simulink model "WindTurbineModel_V2"  (R2025b)
settings: Solver=FixedStepDiscrete  StartTime=0.0  StopTime=inf  FixedStep=.00011  RelTol=1e-3  EnableMultiTasking=on
model workspace (MAT data in the model file):
  lambda = 10
  rho = 1.125
libraries: simulink x4, arduinolib x2, arduinosensorlib x1, slpidlib x1
settings Model: SimulationMode=external  ExtModeTrigDuration=2  Creator=Patron  LastModifiedBy=WEI
settings SolverCC: AllowMultiTaskInputOutput=on  ConcurrentTasks=on  AlgebraicLoopSolver=TrustRegion  AutoInsertRateTranBlk=on  DecoupledContinuousIntegration=on  MinimalZcImpactIntegration=on
settings DataIOCC: ReturnWorkspaceOutputs=off
settings OptimizationCC: EnhancedBackFolding=on  BooleansAsBitfields=on  PassReuseOutputArgsAs=Individual arguments  StateBitsets=on  DataBitsets=on  ZeroExternalMemoryAtStartup=off  ZeroInternalMemoryAtStartup=off  MaxStackSize=64  DifferentSizesBufferReuse=on  OptimizationPriority=RAM  OptimizationCustomize=off  EfficientTunableParamExpr=on
settings DebuggingCC: ParameterTunabilityLossMsg=error  UnconnectedInputMsg=warning  UnconnectedOutputMsg=warning  UnconnectedLineMsg=warning  ArithmeticOperatorsInVariantConditions=warning
settings HardwareCC: ProdBitPerInt=16.0  ProdBitPerPointer=16.0  ProdBitPerSizeT=16.0  ProdBitPerPtrDiffT=16.0  ProdLargestAtomicFloat=None  ProdWordSize=8.0  ProdHWDeviceType=Atmel->AVR
settings ModelReferenceCC: EnableRefExpFcnMdlSchedulingChecks=on
settings SFSimCC: SimUseLocalCustomCode=off  MATLABDynamicMemAlloc=off  CustomCodeUndefinedFunction=UseInterfaceOnly
settings RTWCC: SystemTargetFile=ert.tlc  HardwareBoard=Arduino Uno  TemplateMakefile=ert_default_tmf  RTWUseLocalCustomCode=off  Toolchain=Arduino AVR  BuildConfiguration=Faster Runs  GPUComputeCapability=3.5  DLArmComputeVersion=19.05  Description=Embedded Coder
settings CodeAppCC: ForceParamTrailComments=on  IgnoreCustomStorageClasses=off  MaxIdLength=95.0  OperatorAnnotations=on  SimulinkDataObjDesc=on  SFDataObjDesc=on  InsertBlockDesc=on
settings ERTTargetCC: ExtModeTransport=3.0  ExtModeStaticAlloc=on  ExtModeAutomaticAllocSize=off  ExtModeStaticAllocSize=250.0  ExtModeMexFile=ext_xcp  ExtModeIntrfLevel=Level2 - Open  InlinedParameterPlacement=Hierarchical  SupportContinuousTime=on  SupportVariableSizeSignals=on

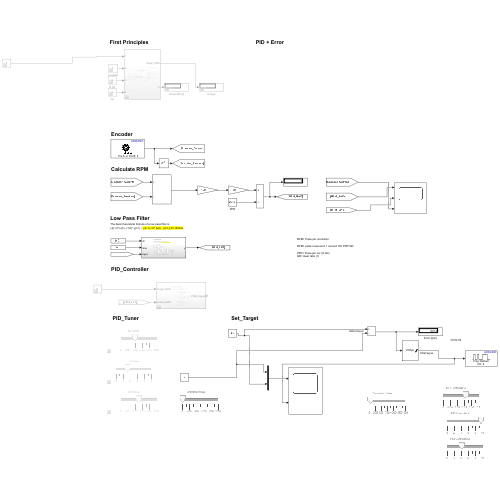
[thumbnail: Simulink's stored preview of the top-level diagram]
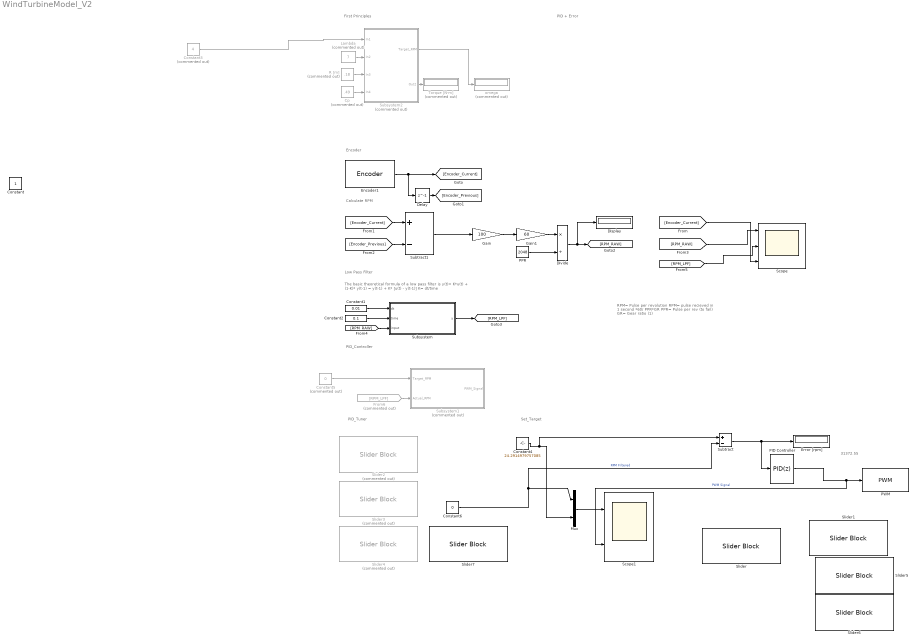
== system WindTurbineModel_V2 ==
  note: PID_Controller
  note: PID + Error
  note: First Principles
  note: The basic theoretical formula of a low pass filter is
      | y(t)= K*u(t) + (1-K)* y(t-1) = y(t-1) + K* [u(t) - y(t-1)] K= dt/time
  note: Low Pass Filter
  note: RPM= Pulse per revolution
      |
      | RPM= pulse recieved in 1 second *60/ PPR*GR
      |
      | PPR= Pulse per rev (to fail)
      | GR= Gear ratio (1)
  note: Calculate RPM
  note: Encoder
  note: PID_Tuner
  note: Set_Target
  note: 31372.55
  Constant1 : Constant  Value=0.01
  Constant2 : Constant  Value=0.1
  Constant3 : Constant  Commented=on  Value=4
  Constant4 : Constant  Value=24.2914979757085
  Constant5 : Constant  Commented=on  Value=0
  Constant6 : Constant  Value=0
  Cp : Constant  Commented=on  Value=.49
  Delay : Delay  DelayLength=1
  Display : Display
  Divide : Product  Inputs=*/
  Encoder1 : arduinosensorlib/Encoder  InputA=2  InputB=3  Mode=No reset  SampleTime=-1
  Error [rpm] : Display
  From6 : From  Commented=on  GotoTag=RPM_LPF
  Gain : Gain  Gain=100
  Gain1 : Gain  Gain=60
  Lambda : Constant  Commented=on  Value=7
  Mux : Mux  Inputs=2
  PID Controller : slpidlib/PID Controller  Controller=PID  Form=Parallel  TimeDomain=Discrete-time  UseExternalTs=off  SampleTime=-1  IntegratorMethod=Forward Euler  FilterMethod=Forward Euler  ControllerParametersSource=internal  P=0.1286549707602339  I=9.534412955465587  UseKiTs=off  D=4.181286549707602  UseExternalDerivativeSource=off  N=100  UseFilter=on  TunerSelectOption=Frequency Response Based  InitialConditionSource=internal  InitialConditionForIntegrator=0  InitialConditionForFilter=0  DifferentiatorICPrevScaledInput=0  ExternalReset=none  TrackingMode=off  Kt=1  LimitOutput=on  SatLimitsSource=internal  UpperSaturationLimit=255  LowerSaturationLimit=0  LinearizeAsGain=on  AntiWindupMode=none  Kb=1  LimitIntegrator=off  UpperIntegratorSaturationLimit=inf  LowerIntegratorSaturationLimit=-inf  POutMin=[]  POutMax=[]  IOutMin=[]  IOutMax=[]  DOutMin=[]  DOutMax=[]  NOutMin=[]  NOutMax=[]  SumOutMin=[]  SumOutMax=[]  SaturationOutMin=[]  SaturationOutMax=[]  PParamMin=[]  PParamMax=[]  IParamMin=[]  IParamMax=[]  DParamMin=[]  DParamMax=[]  NParamMin=[]  NParamMax=[]  KbParamMin=[]  KbParamMax=[]  KtParamMin=[]  KtParamMax=[]  KbOutMin=[]  KbOutMax=[]  KtOutMin=[]  KtOutMax=[]  IntegratorOutMin=[]  IntegratorOutMax=[]  FilterOutMin=[]  FilterOutMax=[]  SumI1OutMin=[]  SumI1OutMax=[]  SumI2OutMin=[]  SumI2OutMax=[]  SumI3OutMin=[]  SumI3OutMax=[]  SumI4OutMin=[]  SumI4OutMax=[]  SumDOutMin=[]  SumDOutMax=[]  DifferentiatorOutMin=[]  DifferentiatorOutMax=[]  FilterDiffOutCoefMin=[]  FilterDiffOutCoefMax=[]  ReciprocalOutMin=[]  ReciprocalOutMax=[]  SumDenOutMin=[]  SumDenOutMax=[]  SumNumOutMin=[]  SumNumOutMax=[]  DivideOutMin=[]  DivideOutMax=[]  UdiffTsProdOutMin=[]  UdiffTsProdOutMax=[]  NTsProdOutMin=[]  NTsProdOutMax=[]  UintegralTsProdOutMin=[]  UintegralTsProdOutMax=[]  UngainTsProdOutMin=[]  UngainTsProdOutMax=[]  ClampingZeroOutDataTypeStr=Inherit: Inherit via back propagation  ClampingZeroOutMin=[]  ClampingZeroOutMax=[]  FilterDenConstantOutDataTypeStr=Inherit: Inherit via back propagation  FilterDenConstantOutMin=[]  FilterDenConstantOutMax=[]  PCopyOutDataTypeStr=Inherit: Inherit via back propagation  PCopyOutMin=[]  PCopyOutMax=[]  NCopyOutDataTypeStr=Inherit: Inherit via back propagation  NCopyOutMin=[]  NCopyOutMax=[]  IntegratorContinuousStateAttributes=''  IntegratorStateMustResolveToSignalObject=off  IntegratorRTWStateStorageClass=Auto  FilterContinuousStateAttributes=''  FilterStateMustResolveToSignalObject=off  FilterRTWStateStorageClass=Auto  ParallelPVariant=InternalParameters  IdealPVariant=Disabled  IVariant=InternalParameters  DVariant=InternalParameters  IntegratorVariant=Discrete  SatVariant=Enabled  AWVariant=Passthrough  PCopyVariant=Disabled  TRVariant=Disabled  FdbkBlocksVariant=Forward  IdealPFdbkVariant=Disabled  SatFdbkVariant=Disabled  DerivativeFilterVariant=ForwardEulerFilter  NVariant=InternalParameters  NCopyVariant=Disabled  FilterICVariant=InternalICsFilter  IntegratorICVariant=InternalICs  ExternalResetVariant=Disabled  TRSumVariant=Passthrough  SumFdbkVariant=Disabled  SumVariant=Sum_PID  TsampFilterVariant=InternalTs  TsampNgainVariant=Passthrough  TsampIntegralVariant=Disabled_SignalSpec  ExternalSaturationOutDataTypeStr=Inherit: Same as second input  DerivativeSourceVariant=ErrorSignal  PreIntVariant=InternalPreInt
  PPR : Constant  Value=2048
  PWM : arduinolib/PWM  pinNumber=9  frequencyType=Default  desiredFrequency=3000  achievableFrequency=2999.625
  R [m] : Constant  Commented=on  Value=.18
  Scope : Scope  NumInputPorts=3
      settings: ActiveDisplayYMinimum=-111615.35287433089  ActiveDisplayYMaximum=303387.53308712941
  Scope1 : Scope  NumInputPorts=2
      settings: ActiveDisplayYMinimum=-159.80323832172013  ActiveDisplayYMaximum=288.71002139995966
  Slider : SliderBlock  ScaleMax=1500
  Slider1 : SliderBlock  ScaleMax=0.2
  Slider2 : SliderBlock  Commented=on  ScaleMax=0.05
  Slider3 : SliderBlock  Commented=on  ScaleMax=5
  Slider4 : SliderBlock  Commented=on  ScaleMax=0.05
  Slider5 : SliderBlock  ScaleMax=10
  Slider6 : SliderBlock  ScaleMax=10
  Slider7 : SliderBlock  ScaleMax=2000
  Subsystem : Subsystem
  Subsystem1 : Subsystem  Commented=on
  Subsystem2 : Subsystem  Commented=on
  Subtract : Sum  Inputs=+-
  Subtract1 : Sum  Inputs=+-
  Torque [N-m] : Display  Commented=on
  omega : Display  Commented=on
  Constant : Constant  IOType=siggen
  wires:
  Subsystem2/1(Target_RPM) -> omega/1
  Constant3/1 -> Subsystem2/1(In1)
  Lambda/1 -> Subsystem2/2(In2)
  R [m]/1 -> Subsystem2/3(In3)
  Cp/1 -> Subsystem2/4(In4)
  Subsystem2/2(Out2) -> Torque [N-m]/1
  Encoder1/1 -> Delay/1, [Encoder_Current]
  [Encoder_Current] -> Scope/3
  Delay/1 -> [Encoder_Previous]
  [Encoder_Current] -> Subtract1/1
  [Encoder_Previous] -> Subtract1/2
  Subtract1/1 -> Gain/1
  Gain/1 -> Gain1/1
  Gain1/1 -> Divide/1
  PPR/1 -> Divide/2
  Divide/1 -> Display/1, [RPM_RAW]
  [RPM_RAW] -> Scope/1
  [RPM_RAW] -> Subsystem/3(input)
  Constant1/1 -> Subsystem/1(dt)
  Constant2/1 -> Subsystem/2(time)
  Subsystem/1(y) -> [RPM_LPF]
  [RPM_LPF] -> Scope/2
  From6/1 -> Subsystem1/2(Actual_RPM)
  PID Controller/1 -> Scope1/2, PWM/1  "PWM Signal"
  Constant6/1 -> Subtract/2, Mux/1  "RPM Filtered"
  Mux/1 -> Scope1/1
  Subtract/1 -> Error [rpm]/1, PID Controller/1
  Constant4/1 -> Subtract/1, Mux/2
  Constant5/1 -> Subsystem1/1(Target_RPM)

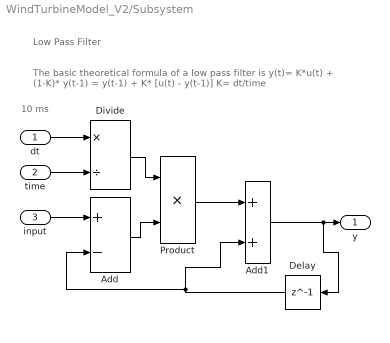
== system WindTurbineModel_V2/Subsystem ==
  note: 10 ms
  note: Low Pass Filter
  note: The basic theoretical formula of a low pass filter is
      | y(t)= K*u(t) + (1-K)* y(t-1) = y(t-1) + K* [u(t) - y(t-1)] K= dt/time
  dt : Inport
  time : Inport  Port=2
  input : Inport  Port=3
  Add : Sum  Inputs=+-
  Add1 : Sum
  Delay : Delay  DelayLength=1
  Divide : Product  Inputs=*/
  Product : Product
  y : Outport
  wires:
  dt/1 -> Divide/1
  time/1 -> Divide/2
  input/1 -> Add/1
  Add/1 -> Product/2
  Divide/1 -> Product/1
  Product/1 -> Add1/1
  Add1/1 -> Delay/1, y/1
  Delay/1 -> Add/2, Add1/2

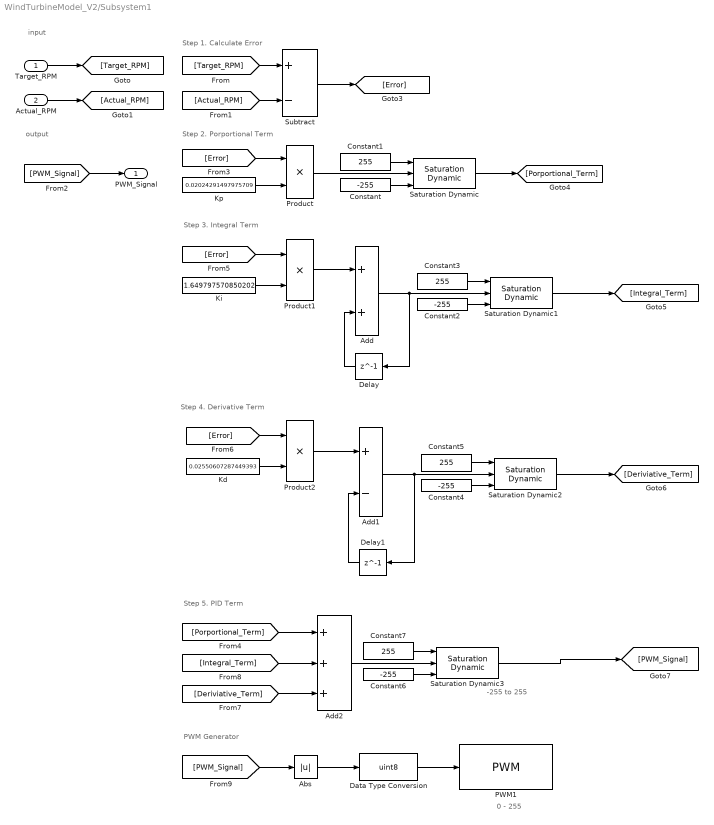
== system WindTurbineModel_V2/Subsystem1 ==
  note: 0 - 255
  note: -255 to 255
  note: Step 2. Porportional Term
  note: output
  note: input
  note: Step 1. Calculate Error
  note: Step 3. Integral Term
  note: Step 4. Derivative Term
  note: Step 5. PID Term
  note: PWM Generator
  Target_RPM : Inport
  Actual_RPM : Inport  Port=2
  Abs : Abs  SaturateOnIntegerOverflow=off
  Add : Sum
  Add1 : Sum  Inputs=+-
  Add2 : Sum  Inputs=+++
  Constant{,2,4,6} (4 alike) : Constant  Value=-255
  Constant{1,3,5,7} (4 alike) : Constant  Value=255
  Data Type Conversion : DataTypeConversion  OutMin=0  OutMax=255  OutDataTypeStr=uint8  SaturateOnIntegerOverflow=off  RndMeth=Floor
  Delay : Delay  DelayLength=1
  Delay1 : Delay  DelayLength=1
  Kd : Constant  Value=0.02550607287449393
  Ki : Constant  Value=1.649797570850202
  Kp : Constant  Value=0.02024291497975709
  PWM1 : arduinolib/PWM  pinNumber=9  frequencyType=Default  desiredFrequency=3921.16  achievableFrequency=3921.5686
  Product : Product
  Product1 : Product
  Product2 : Product
  Saturation Dynamic{,1..3} (4 alike) : simulink/Discontinuities/Saturation Dynamic  OutMin=[]  OutMax=[]  OutDataTypeStr=Inherit: Same as second input  OutDataType=fixdt(1, 16)  OutScaling=2^-10  DoSatur=off
  Subtract : Sum  Inputs=+-
  PWM_Signal : Outport
  wires:
  Target_RPM/1 -> [Target_RPM]
  Actual_RPM/1 -> [Actual_RPM]
  [PWM_Signal] -> PWM_Signal/1
  [Actual_RPM] -> Subtract/2
  [Target_RPM] -> Subtract/1
  Subtract/1 -> [Error]
  Kp/1 -> Product/2
  [Error] -> Product/1
  [Error] -> Product1/1
  Ki/1 -> Product1/2
  Product/1 -> Saturation Dynamic/2
  Product1/1 -> Add/1
  Add/1 -> Saturation Dynamic1/2, Delay/1
  Delay/1 -> Add/2
  [Error] -> Product2/1
  Kd/1 -> Product2/2
  Product2/1 -> Add1/1
  Add1/1 -> Saturation Dynamic2/2, Delay1/1
  Delay1/1 -> Add1/2
  [Deriviative_Term] -> Add2/3
  [Integral_Term] -> Add2/2
  [Porportional_Term] -> Add2/1
  Add2/1 -> Saturation Dynamic3/2
  [PWM_Signal] -> Abs/1
  Data Type Conversion/1 -> PWM1/1
  Abs/1 -> Data Type Conversion/1
  Saturation Dynamic3/1 -> [PWM_Signal]
  Saturation Dynamic2/1 -> [Deriviative_Term]
  Saturation Dynamic1/1 -> [Integral_Term]
  Saturation Dynamic/1 -> [Porportional_Term]
  Constant/1 -> Saturation Dynamic/3
  Constant1/1 -> Saturation Dynamic/1
  Constant2/1 -> Saturation Dynamic1/3
  Constant3/1 -> Saturation Dynamic1/1
  Constant4/1 -> Saturation Dynamic2/3
  Constant5/1 -> Saturation Dynamic2/1
  Constant6/1 -> Saturation Dynamic3/3
  Constant7/1 -> Saturation Dynamic3/1

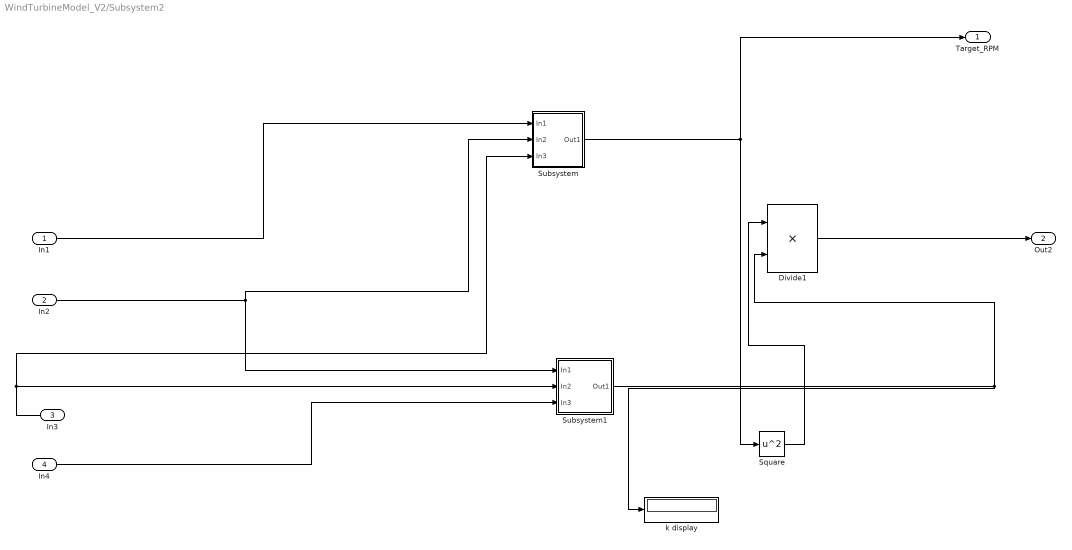
== system WindTurbineModel_V2/Subsystem2 ==
  In1 : Inport
  In2 : Inport  Port=2
  In3 : Inport  Port=3
  In4 : Inport  Port=4
  Divide1 : Product  Inputs=**
  Square : Math  Operator=square
  Subsystem : Subsystem
  Subsystem1 : Subsystem
  k display : Display
  Target_RPM : Outport
  Out2 : Outport  Port=2
  wires:
  Subsystem/1(Out1) -> Target_RPM/1, Square/1
  In3/1 -> Subsystem1/2(In2), Subsystem/3(In3)
  In4/1 -> Subsystem1/3(In3)
  In2/1 -> Subsystem1/1(In1), Subsystem/2(In2)
  Square/1 -> Divide1/1
  Divide1/1 -> Out2/1
  Subsystem1/1(Out1) -> k display/1, Divide1/2
  In1/1 -> Subsystem/1(In1)

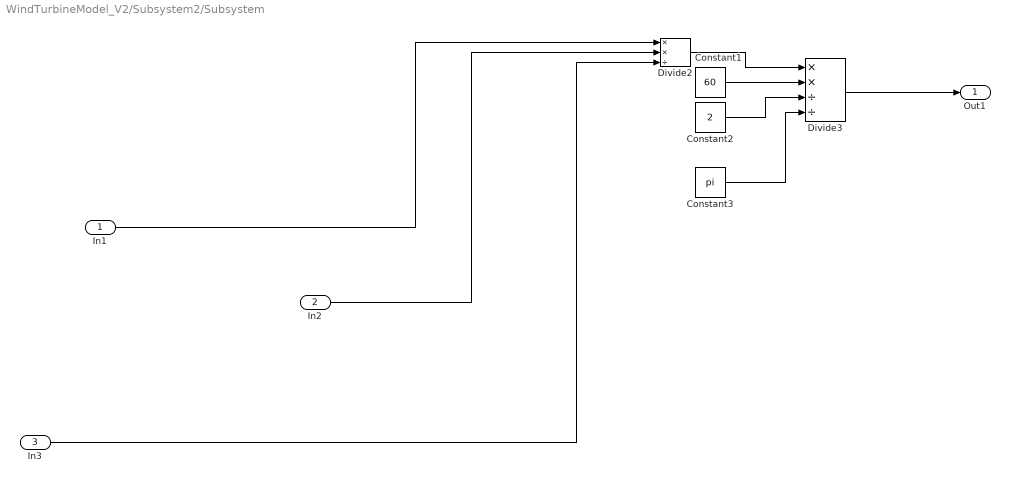
== system WindTurbineModel_V2/Subsystem2/Subsystem ==
  In1 : Inport
  In2 : Inport  Port=2
  In3 : Inport  Port=3
  Constant1 : Constant  Value=60
  Constant2 : Constant  Value=2
  Constant3 : Constant  Value=pi
  Divide2 : Product  Inputs=**/
  Divide3 : Product  Inputs=**//
  Out1 : Outport
  wires:
  Divide3/1 -> Out1/1
  Constant1/1 -> Divide3/2
  In1/1 -> Divide2/1
  Constant3/1 -> Divide3/4
  Divide2/1 -> Divide3/1
  Constant2/1 -> Divide3/3
  In2/1 -> Divide2/2
  In3/1 -> Divide2/3

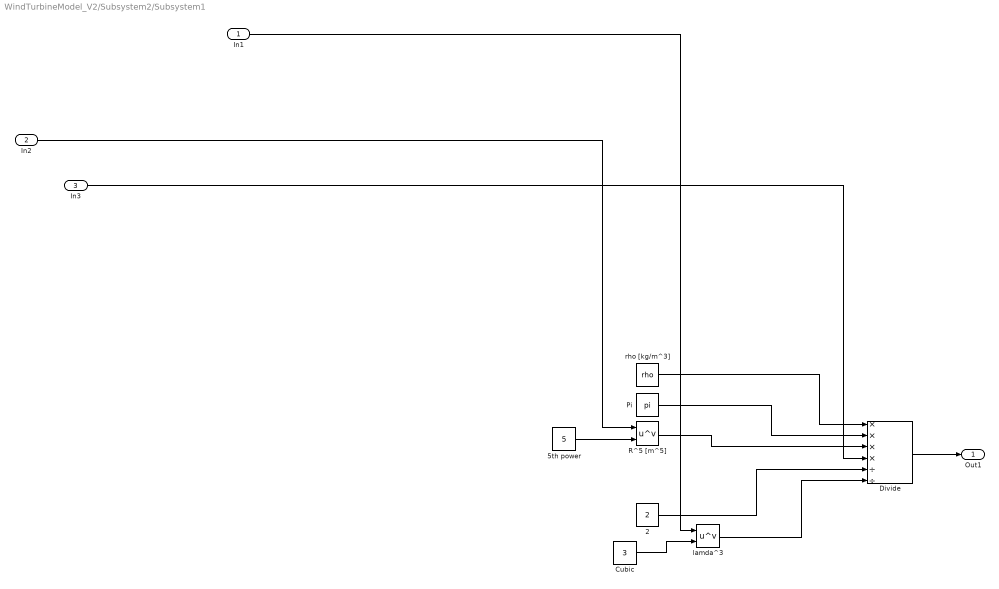
== system WindTurbineModel_V2/Subsystem2/Subsystem1 ==
  In1 : Inport
  In2 : Inport  Port=2
  In3 : Inport  Port=3
  2 : Constant  Value=2
  5th power : Constant  Value=5
  Cubic : Constant  Value=3
  Divide : Product  Inputs=****//
  Pi : Constant  Value=pi  OutDataTypeStr=Inherit: Inherit via back propagation
  R^5 [m^5] : Math  Operator=pow
  lamda^3 : Math  Operator=pow
  rho [kg/m^3] : Constant  Value=rho
  Out1 : Outport
  wires:
  lamda^3/1 -> Divide/6
  rho [kg/m^3]/1 -> Divide/1
  In1/1 -> lamda^3/1
  5th power/1 -> R^5 [m^5]/2
  In3/1 -> Divide/4
  Pi/1 -> Divide/2
  R^5 [m^5]/1 -> Divide/3
  2/1 -> Divide/5
  In2/1 -> R^5 [m^5]/1
  Cubic/1 -> lamda^3/2
  Divide/1 -> Out1/1
